simulink model "thursterVariable"  (R2023a)
settings: Solver=ode4  StartTime=0.0  StopTime=10.0  FixedStep=dt  RelTol=1e-3
settings Model: Creator=hugobuurmeijer  LastModifiedBy=ndelurgio

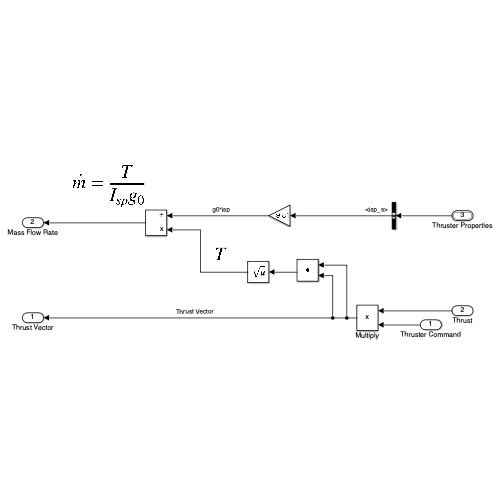
[thumbnail: Simulink's stored preview of the top-level diagram]
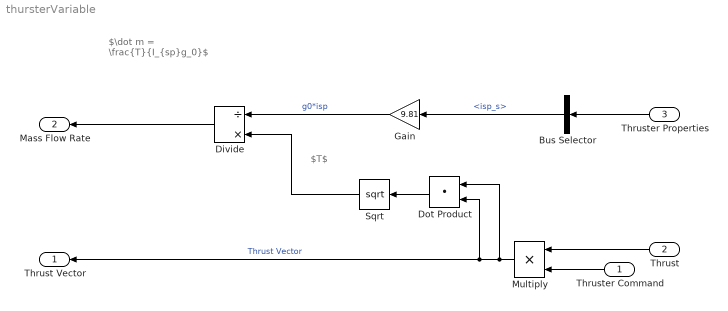
== system thursterVariable ==
  note: $T$
  note: $\dot m = \frac{T}{I_{sp}g_0}$
  Thruster Command : Inport
  Thrust : Inport  Port=2  PortDimensions=3
  Thruster Properties : Inport  Port=3  OutDataTypeStr=Bus: thruster
  Bus Selector : BusSelector  OutputSignals=isp_s
  Divide : Product  Inputs=/*
  Dot Product : DotProduct  InputSameDT=off  OutDataTypeStr=Inherit: Inherit via internal rule
  Gain : Gain  Gain=9.81
  Multiply : Product  Inputs=**
  Sqrt : Sqrt
  Thrust Vector : Outport  PortDimensions=3
  Mass Flow Rate : Outport  Port=2
  wires:
  Thruster Properties/1 -> Bus Selector/1
  Gain/1 -> Divide/1  "g0*isp"
  Divide/1 -> Mass Flow Rate/1
  Thrust/1 -> Multiply/1
  Multiply/1 -> Dot Product/1, Dot Product/2, Thrust Vector/1  "Thrust Vector"
  Bus Selector/1 -> Gain/1  "<isp_s>"
  Thruster Command/1 -> Multiply/2
  Dot Product/1 -> Sqrt/1
  Sqrt/1 -> Divide/2
